simulink subsystem "PvtSubSys_VSM_HWA"  (R2020b)
settings: Solver=VariableStepAuto  StartTime=0.0  StopTime=10.0  RelTol=1e-3
values from neighbouring files (symbols this model uses):
  P_VSM_HWA_ALCStsSW = 1    [HWA.sldd]
  P_VSM_HWA_DMS_Enable = 0.0    [HWA.sldd]
  P_VSM_HWA_EHR_Enable = 0.0    [HWA.sldd]
  P_VSM_HWAActivation_NOAMOd_Spd = 5.0    [HWA.sldd]
  P_VSM_HWAActivation_Spd_Low = 5.0    [HWA.sldd]
  P_VSM_HWAActivation_Spd_Up = 120.0    [HWA.sldd]
  P_VSM_NOH_PilotSelc_SW = 0.0    [HWA.sldd]
  P_VSM_NOH_Swt_Req_SW = 0.0    [HWA.sldd]
  P_VSM_TJA_PassSBRSpdExistSlow = 30.0    [HWA.sldd]
undefined symbols (not defined in the file or in its folder): ACC_STATE, P_VSM_PassSBRSpdIPLimt, TJA_STATE
libraries: simulink x65, TrueDurationTime x14
(part 1 of 2)
settings Model: Creator=GW00133806  LastModifiedBy=GW00201299

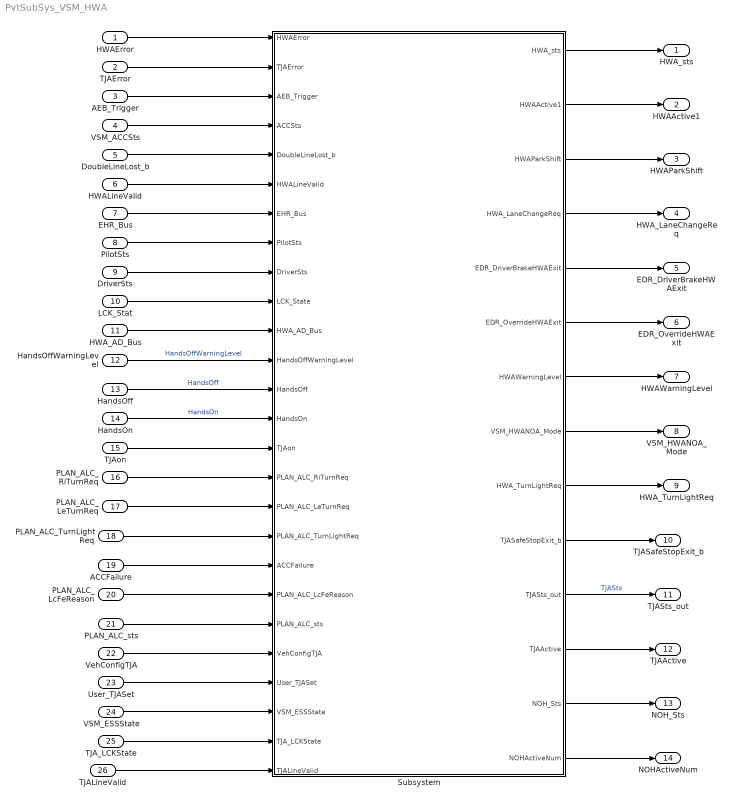
== system PvtSubSys_VSM_HWA ==
  HWAError : Inport  OutDataTypeStr=uint8
  TJAError : Inport  Port=2
  AEB_Trigger : Inport  Port=3  OutDataTypeStr=boolean
  VSM_ACCSts : Inport  Port=4  OutDataTypeStr=Enum: ACC_STATE
  DoubleLineLost_b : Inport  Port=5  OutDataTypeStr=boolean
  HWALineValid : Inport  Port=6  OutDataTypeStr=boolean
  EHR_Bus : Inport  Port=7  OutDataTypeStr=Bus: EHR_Bus
  PilotSts : Inport  Port=8  OutDataTypeStr=uint8
  DriverSts : Inport  Port=9  OutDataTypeStr=uint8
  LCK_Stat : Inport  Port=10
  HWA_AD_Bus : Inport  Port=11
  HandsOffWarningLevel : Inport  Port=12  OutDataTypeStr=uint8
  HandsOff : Inport  Port=13  OutDataTypeStr=boolean
  HandsOn : Inport  Port=14  OutDataTypeStr=boolean
  TJAon : Inport  Port=15  OutDataTypeStr=boolean
  PLAN_ALC_RiTurnReq : Inport  Port=16  OutDataTypeStr=uint8
  PLAN_ALC_LeTurnReq : Inport  Port=17  OutDataTypeStr=uint8
  PLAN_ALC_TurnLightReq : Inport  Port=18  OutDataTypeStr=uint8
  ACCFailure : Inport  Port=19
  PLAN_ALC_LcFeReason : Inport  Port=20
  PLAN_ALC_sts : Inport  Port=21
  VehConfigTJA : Inport  Port=22
  User_TJASet : Inport  Port=23
  VSM_ESSState : Inport  Port=24
  TJA_LCKState : Inport  Port=25
  TJALineValid : Inport  Port=26
  Subsystem : Subsystem
  HWA_sts : Outport  OutDataTypeStr=Enum: HWA_STATE
  HWAActive1 : Outport  Port=2  OutDataTypeStr=boolean
  HWAParkShift : Outport  Port=3  OutDataTypeStr=boolean
  HWA_LaneChangeReq : Outport  Port=4  OutDataTypeStr=uint8
  EDR_DriverBrakeHWAExit : Outport  Port=5  OutDataTypeStr=boolean
  EDR_OverrideHWAExit : Outport  Port=6  OutDataTypeStr=boolean
  HWAWarningLevel : Outport  Port=7  OutDataTypeStr=uint8
  VSM_HWANOA_Mode : Outport  Port=8  OutDataTypeStr=uint8
  HWA_TurnLightReq : Outport  Port=9
  TJASafeStopExit_b : Outport  Port=10
  TJASts_out : Outport  Port=11
  TJAActive : Outport  Port=12
  NOH_Sts : Outport  Port=13
  NOHActiveNum : Outport  Port=14
  wires:
  TJAError/1 -> Subsystem/2(TJAError)
  PLAN_ALC_sts/1 -> Subsystem/21(PLAN_ALC_sts)
  ACCFailure/1 -> Subsystem/19(ACCFailure)
  Subsystem/9(HWA_TurnLightReq) -> HWA_TurnLightReq/1
  PLAN_ALC_TurnLightReq/1 -> Subsystem/18(PLAN_ALC_TurnLightReq)
  Subsystem/8(VSM_HWANOA_Mode) -> VSM_HWANOA_Mode/1
  HandsOff/1 -> Subsystem/13(HandsOff)  "HandsOff"
  AEB_Trigger/1 -> Subsystem/3(AEB_Trigger)
  Subsystem/7(HWAWarningLevel) -> HWAWarningLevel/1
  Subsystem/5(EDR_DriverBrakeHWAExit) -> EDR_DriverBrakeHWAExit/1
  HWALineValid/1 -> Subsystem/6(HWALineValid)
  PilotSts/1 -> Subsystem/8(PilotSts)
  VSM_ACCSts/1 -> Subsystem/4(ACCSts)
  EHR_Bus/1 -> Subsystem/7(EHR_Bus)
  TJAon/1 -> Subsystem/15(TJAon)
  DoubleLineLost_b/1 -> Subsystem/5(DoubleLineLost_b)
  Subsystem/3(HWAParkShift) -> HWAParkShift/1
  Subsystem/2(HWAActive1) -> HWAActive1/1
  HandsOn/1 -> Subsystem/14(HandsOn)  "HandsOn"
  HWA_AD_Bus/1 -> Subsystem/11(HWA_AD_Bus)
  Subsystem/1(HWA_sts) -> HWA_sts/1
  PLAN_ALC_LeTurnReq/1 -> Subsystem/17(PLAN_ALC_LeTurnReq)
  LCK_Stat/1 -> Subsystem/10(LCK_State)
  DriverSts/1 -> Subsystem/9(DriverSts)
  HWAError/1 -> Subsystem/1(HWAError)
  Subsystem/6(EDR_OverrideHWAExit) -> EDR_OverrideHWAExit/1
  HandsOffWarningLevel/1 -> Subsystem/12(HandsOffWarningLevel)  "HandsOffWarningLevel"
  Subsystem/4(HWA_LaneChangeReq) -> HWA_LaneChangeReq/1
  PLAN_ALC_RiTurnReq/1 -> Subsystem/16(PLAN_ALC_RiTurnReq)
  PLAN_ALC_LcFeReason/1 -> Subsystem/20(PLAN_ALC_LcFeReason)
  VehConfigTJA/1 -> Subsystem/22(VehConfigTJA)
  User_TJASet/1 -> Subsystem/23(User_TJASet)
  VSM_ESSState/1 -> Subsystem/24(VSM_ESSState)
  TJA_LCKState/1 -> Subsystem/25(TJA_LCKState)
  TJALineValid/1 -> Subsystem/26(TJALineValid)
  Subsystem/10(TJASafeStopExit_b) -> TJASafeStopExit_b/1
  Subsystem/11(TJASts_out) -> TJASts_out/1  "TJASts"
  Subsystem/12(TJAActive) -> TJAActive/1
  Subsystem/13(NOH_Sts) -> NOH_Sts/1
  Subsystem/14(NOHActiveNum) -> NOHActiveNum/1

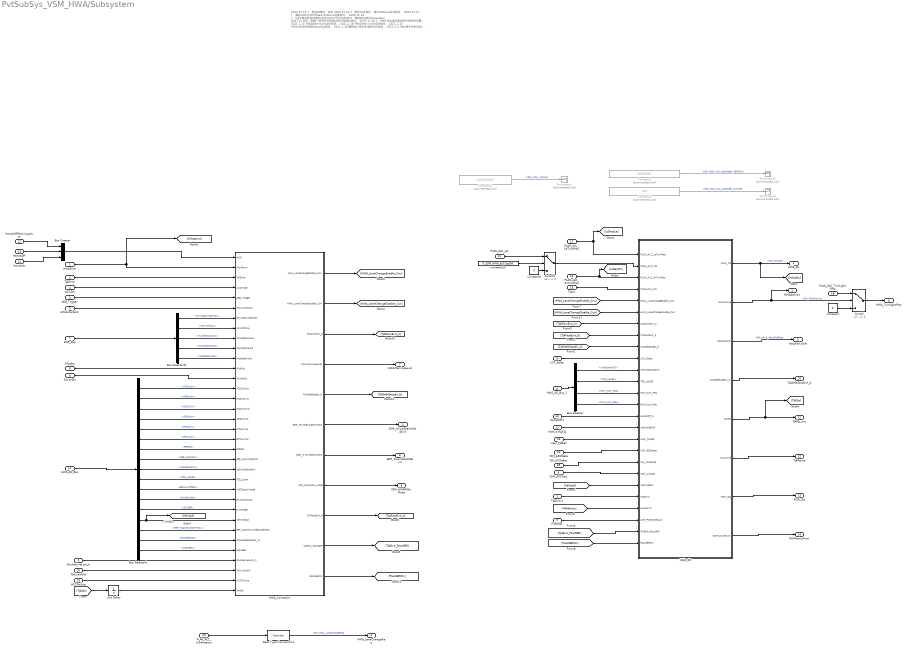
== system PvtSubSys_VSM_HWA/Subsystem ==
  note: 2020.12.15
      | 1、新框架释放，初版
      |
      | 2020.12.16
      | 1、更新NOA条件，增加NOAmode观测点；
      | 2020.12.17
      | 1、删除HWA状态机Ready到Active速度条件。
      | 2020.12.18
      | 1、HWA慢退进快退增加HWA状态处于CC校验条件，慢退条件满足且Handson
      |       且处于CC状态，屏蔽一些条件在换道过程中导致的退出。
      | 2020.12.28
      | 1. HWA 状态激活速度条件做成标定量。
      | 2021.1.15
      | HWAWarning状态机修改；
      | 2021.1.18
      | HWAWarning状态机修改；
      | 2021.1.19
      | HWA状态机换道信号coding修改；
      | 2021.1.20
      | 删除进入条件车速的时间校验；
      | 2021.2.2
      | HWA脱手条件连接。
      | 2021.2.5
      | HWA进慢退逻辑修改
      | 2021.2.6
      | 进慢退逻辑修改
      | 2021.2.8
      | 增加观测量；
      | 2021.2.17
      | 增加慢退条件ACCError
      | HWA状态机Error修改；
      | 2021.2.22
      | HWA_LaneChangeReq修改；
      | 接口修改；
      | 2021.2.26
      | 因PLAN版本未变更，断开ALCSts；
      | 2021.3.4
      | HWADriveOffConds修改HWA无法起步问题；
      | 2021.3.12
      | SafeStop置位延迟5s
      | 2021.3.13
      | 修改HWA跟停起步退出问题；
      | 解决HWA未激活报HWA_Warning的问题；
      | 2021.3.16
      | SingleLineLost进入慢退时加延时，增加标定量P_VSM_HWASlowExit_SingleLineLostDuring，默认3s；
  HWAError : Inport  OutDataTypeStr=uint8
  TJAError : Inport  Port=2
  AEB_Trigger : Inport  Port=3  OutDataTypeStr=boolean
  ACCSts : Inport  Port=4  OutDataTypeStr=Enum: ACC_STATE
  DoubleLineLost_b : Inport  Port=5
  HWALineValid : Inport  Port=6  OutDataTypeStr=boolean
  EHR_Bus : Inport  Port=7  OutDataTypeStr=Bus: EHR_Bus
  PilotSts : Inport  Port=8  OutDataTypeStr=uint8
  DriverSts : Inport  Port=9  OutDataTypeStr=uint8
  LCK_State : Inport  Port=10
  HWA_AD_Bus : Inport  Port=11
  HandsOffWarningLevel : Inport  Port=12  OutDataTypeStr=uint8
  HandsOff : Inport  Port=13  OutDataTypeStr=boolean
  HandsOn : Inport  Port=14  OutDataTypeStr=boolean
  TJAon : Inport  Port=15  OutDataTypeStr=boolean
  PLAN_ALC_RiTurnReq : Inport  Port=16  OutDataTypeStr=uint8
  PLAN_ALC_LeTurnReq : Inport  Port=17  OutDataTypeStr=uint8
  PLAN_ALC_TurnLightReq : Inport  Port=18
  ACCFailure : Inport  Port=19
  PLAN_ALC_LcFeReason : Inport  Port=20
  PLAN_ALC_sts : Inport  Port=21
  VehConfigTJA : Inport  Port=22
  User_TJASet : Inport  Port=23
  VSM_ESSState : Inport  Port=24
  TJA_LCKState : Inport  Port=25
  TJALineValid : Inport  Port=26
  Bus Creator : BusCreator  Inputs=3
  Bus Selector : BusSelector  OutputSignals=VehStandstill,TGS_LEVER,NOH_Swt_Req,NOH_Act_Req
  Bus Selector31 : BusSelector  OutputSignals=DrivingOnHighWay,FormOfWay,TunnelDistance,RampDistance,MapDataValid
  Bus Selector5 : BusSelector  OutputSignals=VDCActv,MSRActv,HDCCtrl,ABSActv,PTCActv,BTCActv,EPBSts,EPB_SwtPosn,VehStandstill,TGS_LEVER,ESPFuncOffSts,DrvDoorSts,DrvSBR,VehSpd,ESP_MasterCylBrkPress,BrkPedalSts,PassSBR
  Constant : Constant  Value=0  OutDataTypeStr=uint8
  Constant1 : Constant  Commented=on  Value=38260536  OutDataTypeStr=uint32
  Constant10 : Constant  Value=P_VSM_HWA_ALCStsSW
  Constant2 : Constant  Commented=on  Value=2103160605
  Constant3 : Constant  Commented=on  Value=301  OutDataTypeStr=uint16
  Constant9 : Constant  Value=0  OutDataTypeStr=uint8
  Data Type Conversion1 : DataTypeConversion
  HWA_AD_Bus_1 : InportShadow  Port=11
  HWA_Condotion : Subsystem
  HWA_SM : Subsystem
  HandsOff1 : InportShadow  Port=13  OutDataTypeStr=boolean
  PilotSts1 : InportShadow  Port=8  OutDataTypeStr=uint8
  Switch : Switch  Criteria=u2 ~= 0
  Switch6 : Switch  Criteria=u2 ~= 0
  TJAError1 : InportShadow  Port=2
  Terminator1 : Terminator  Commented=on
  Terminator2 : Terminator  Commented=on
  Terminator3 : Terminator  Commented=on
  Unit Delay : UnitDelay  InitialCondition=TJA_STATE.TJA_Off  SampleTime=-1  HasFrameUpgradeWarning=on
  VSM_ACCSts1 : InportShadow  Port=4  OutDataTypeStr=Enum: ACC_STATE
  HWA_sts : Outport  OutDataTypeStr=Enum: HWA_STATE
  HWAActive1 : Outport  Port=2  OutDataTypeStr=boolean
  HWAParkShift : Outport  Port=3  OutDataTypeStr=boolean
  HWA_LaneChangeReq : Outport  Port=4  OutDataTypeStr=uint8
  EDR_DriverBrakeHWAExit : Outport  Port=5  OutDataTypeStr=boolean
  EDR_OverrideHWAExit : Outport  Port=6  OutDataTypeStr=boolean
  HWAWarningLevel : Outport  Port=7  OutDataTypeStr=uint8
  VSM_HWANOA_Mode : Outport  Port=8  OutDataTypeStr=uint8
  HWA_TurnLightReq : Outport  Port=9
  TJASafeStopExit_b : Outport  Port=10
  TJASts_out : Outport  Port=11
  TJAActive : Outport  Port=12
  NOH_Sts : Outport  Port=13
  NOHActiveNum : Outport  Port=14
  wires:
  [TJAExit_PassSBR] -> HWA_SM/25(TJAExit_PassSBR)
  [PassSBROn] -> HWA_SM/26(PassSBROn)
  HWA_Condotion/11(PassSBROn) -> [PassSBROn]
  HWA_Condotion/10(TJAExit_PassSBR) -> [TJAExit_PassSBR]
  Bus Selector5/17 -> HWA_Condotion/30("PassSBR ")  "<PassSBR>"
  HWA_SM/8(NOHActiveNum) -> NOHActiveNum/1
  Bus Selector/4 -> HWA_SM/14(NOH_Act_Req)  "<NOH_Act_Req>"
  HWA_SM/7(NOH_Sts) -> NOH_Sts/1
  Bus Selector/3 -> HWA_SM/13(NOH_Swt_Req)  "<NOH_Swt_Req>"
  PilotSts1/1 -> HWA_SM/24(LSM_PilotModeCalc)
  [HWAerror] -> HWA_SM/23(HWAerror)
  HWA_SM/6(TJAActive) -> TJAActive/1
  [VehSpd] -> HWA_SM/21(VehicleSpd)
  Unit Delay/1 -> HWA_Condotion/34(TJASts)
  [TJASts] -> Unit Delay/1
  TJALineValid/1 -> HWA_Condotion/32(TJALineValid)
  DoubleLineLost_b/1 -> HWA_Condotion/31(DoubleLineLost_b)
  TJA_LCKState/1 -> HWA_SM/19(TJA_LCKState)
  VSM_ESSState/1 -> HWA_SM/18(VSM_ESSState)
  User_TJASet/1 -> HWA_SM/17(User_TJASet)
  VehConfigTJA/1 -> HWA_SM/16(VehConfigTJA)
  VSM_ACCSts1/1 -> HWA_SM/20(VSM_ACCSts)
  HandsOff1/1 -> HWA_SM/15(HandsOff_b)
  HWA_SM/5(TJASts) -> TJASts_out/1, [TJASts]
  HWA_SM/4(TJASafeStopExit_b) -> TJASafeStopExit_b/1
  [TJASafeStopEn_b] -> HWA_SM/9(TJASafeStopEn_b)
  [TJAFastExit_b] -> HWA_SM/8(TJAFastExit_b)
  HWA_Condotion/9(TJAFastExit_b) -> [TJAFastExit_b]
  HWALineValid/1 -> HWA_Condotion/6(HWALineValid)
  Bus Selector5/15 -> HWA_Condotion/28(ESP_MasterCylindBrakePress)  "<ESP_MasterCylBrkPress>"
  HWA_SM/1(HWA_sts) -> [HWASts], HWA_sts/1  "VSM_HWASts"
  DriverSts/1 -> HWA_Condotion/13(DriverSts)
  Bus Selector31/1 -> HWA_Condotion/7(DrivingOnHighWay)  "<DrivingOnHighWay>"
  HWA_Condotion/2(HWA_LaneChangeDisable_Con) -> [HWA_LaneChangeDisable_Con]
  Bus Selector5/10 -> HWA_Condotion/23(TGS_Lever)  "<TGS_LEVER>"
  HWA_SM/2(HWAActive) -> Switch/2, HWAActive1/1  "VSM_HWAActive"
  Bus Selector5/3 -> HWA_Condotion/16(HDCControl)  "<HDCCtrl>"
  PilotSts/1 -> HWA_Condotion/12(PilotSts)
  AEB_Trigger/1 -> HWA_Condotion/5(AEB_Trigger)
  Bus Selector5/9 -> HWA_Condotion/22(VehicleStandstill)  "<VehStandstill>"
  PLAN_ALC_RiTurnReq/1 -> HWA_SM/3(PLAN_ALC_RiTurnReq), [LcDecsRi]
  HWA_AD_Bus/1 -> Bus Selector5/1
  Bus Selector5/16 -> HWA_Condotion/29(BrakePedalStatus_G)  "<BrkPedalSts>"
  Bus Selector5/1 -> HWA_Condotion/14(VDCActive)  "<VDCActv>"
  HWA_SM/3(TJAParkShift) -> HWAParkShift/1  "VSM_HWA_ParkShiftReq"
  HWAError/1 -> HWA_Condotion/2(HWAError), [HWAerror]
  Bus Creator/1 -> HWA_Condotion/1(HOD)
  Bus Selector5/7 -> HWA_Condotion/20(EPBSts)  "<EPBSts>"
  HWA_AD_Bus_1/1 -> Bus Selector/1
  [HWA_LaneChangeDisable_Con] -> HWA_SM/6(HWA_LaneChangeDisable_Con)
  HandsOffWarningLevel/1 -> Bus Creator/1
  HWA_Condotion/1(HWA_LaneChangeEnable_Con) -> [HWA_LaneChangeEnable_Con]
  Bus Selector5/2 -> HWA_Condotion/15(MSRActive)  "<MSRActv>"
  [HWA_LaneChangeEnable_Con] -> HWA_SM/5(HWA_LaneChangeEnable_Con)
  Bus Selector5/12 -> HWA_Condotion/25(DriverDoorSts)  "<DrvDoorSts>"
  HWA_Condotion/6(EDR_DriverBrakeHWAExit) -> EDR_DriverBrakeHWAExit/1
  TJAon/1 -> HWA_SM/4(TJASwitch_ON)
  Bus Selector31/4 -> HWA_Condotion/10(RampDistance)  "<RampDistance>"
  EHR_Bus/1 -> Bus Selector31/1
  HandsOff/1 -> Bus Creator/2
  Bus Selector5/11 -> HWA_Condotion/24(VDCDeactivated)  "<ESPFuncOffSts>"
  Bus Selector5/14 -> HWA_Condotion/27(VehicleSpd), [VehSpd]  "<VehSpd>"
  HandsOn/1 -> Bus Creator/3
  HWA_Condotion/4(HWAWarningLevel) -> HWAWarningLevel/1
  Bus Selector5/5 -> HWA_Condotion/18(PTCActive)  "<PTCActv>"
  [TJASlowExit_b] -> HWA_SM/7(TJASlowExit_b)
  HWA_Condotion/3(TJASlowExit_b) -> [TJASlowExit_b]
  Bus Selector5/13 -> HWA_Condotion/26(DriverSBR)  "<DrvSBR>"
  Bus Selector/1 -> HWA_SM/11(VehicleStandstill)  "<VehStandstill>"
  Bus Selector5/4 -> HWA_Condotion/17(ABSActive)  "<ABSActv>"
  Bus Selector31/2 -> HWA_Condotion/8(FormOfWay)  "<FormOfWay>"
  HWA_Condotion/5(TJASafeStopEn_b) -> [TJASafeStopEn_b]
  Bus Selector31/3 -> HWA_Condotion/9(TunnelDistance)  "<TunnelDistance>"
  Bus Selector5/8 -> HWA_Condotion/21(EPB_SwtichPositon)  "<EPB_SwtPosn>"
  Bus Selector5/6 -> HWA_Condotion/19(BTCActive)  "<BTCActv>"
  PLAN_ALC_LeTurnReq/1 -> [LcDecsLe], HWA_SM/1(PLAN_ALC_LeTurnReq)
  Bus Selector31/5 -> HWA_Condotion/11(MapDataValid)  "<MapDataValid>"
  LCK_State/1 -> HWA_SM/10(LCK_State)
  HWA_Condotion/7(EDR_OverrideHWAExit) -> EDR_OverrideHWAExit/1
  ACCSts/1 -> HWA_Condotion/4(ACCMode)
  Data Type Conversion1/1 -> HWA_LaneChangeReq/1  "VSM_HWA_LaneChangeReq"
  HWA_Condotion/8(VSM_HWANOA_Mode) -> VSM_HWANOA_Mode/1
  PLAN_ALC_TurnLightReq/1 -> Switch/1
  Constant/1 -> Switch/3
  Switch/1 -> HWA_TurnLightReq/1
  Constant2/1 -> Terminator1/1  "VSM_HWA_Version"
  ACCFailure/1 -> HWA_Condotion/33(ACCFailure)
  Switch6/1 -> HWA_SM/2(PLAN_ALC_sts)
  Constant10/1 -> Switch6/2
  Constant9/1 -> Switch6/3
  PLAN_ALC_sts/1 -> Switch6/1
  PLAN_ALC_LcFeReason/1 -> Data Type Conversion1/1
  Bus Selector/2 -> HWA_SM/12(TGS_LEVER)  "<TGS_LEVER>"
  TJAError/1 -> HWA_Condotion/3(TJAError)
  TJAError1/1 -> HWA_SM/22(TJAError)
  Constant3/1 -> Terminator3/1  "VSM_HWA_TJA_SubModel_Number"
  Constant1/1 -> Terminator2/1  "VSM_HWA_TJA_SubModel_VERSION"

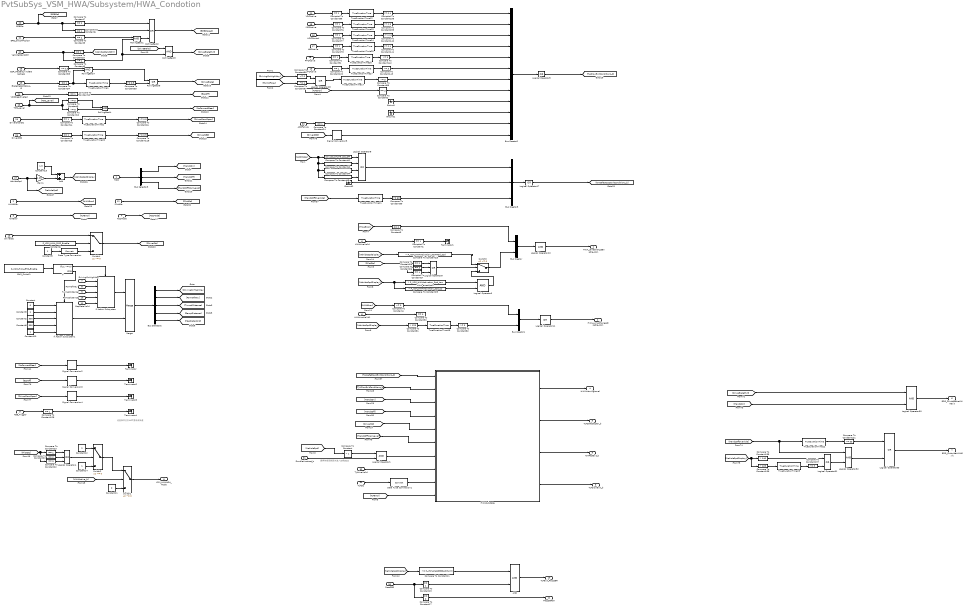
== system PvtSubSys_VSM_HWA/Subsystem/HWA_Condotion ==
  note: 跟停时报双侧丢失进入safestop
  note: 这些条件已在ACC里设成快退
  HOD : Inport
  HWAError : Inport  Port=2
  TJAError : Inport  Port=3
  ACCMode : Inport  Port=4
  AEB_Trigger : Inport  Port=5
  HWALineValid : Inport  Port=6
  DrivingOnHighWay : Inport  Port=7
  FormOfWay : Inport  Port=8
  TunnelDistance : Inport  Port=9
  RampDistance : Inport  Port=10
  MapDataValid : Inport  Port=11
  PilotSts : Inport  Port=12
  DriverSts : Inport  Port=13
  VDCActive : Inport  Port=14
  MSRActive : Inport  Port=15
  HDCControl : Inport  Port=16
  ABSActive : Inport  Port=17
  PTCActive : Inport  Port=18
  BTCActive : Inport  Port=19
  EPBSts : Inport  Port=20
  EPB_SwtichPositon : Inport  Port=21
  VehicleStandstill : Inport  Port=22
  TGS_Lever : Inport  Port=23
  VDCDeactivated : Inport  Port=24
  DriverDoorSts : Inport  Port=25
  DriverSBR : Inport  Port=26
  VehicleSpd : Inport  Port=27
  ESP_MasterCylindBrakePress : Inport  Port=28
  BrakePedalStatus_G : Inport  Port=29
  "PassSBR " : Inport  Port=30
  DoubleLineLost_b : Inport  Port=31
  TJALineValid : Inport  Port=32
  ACCFailure : Inport  Port=33
  TJASts : Inport  Port=34
  AND : Logic  AllPortsSameDT=off  OutDataTypeStr=boolean
  Add : Sum
  Bus Creator : BusCreator  Inputs=2
  Bus Creator1 : BusCreator  Inputs=2
  Bus Creator5 : BusCreator  Inputs=3
  Bus Selector2 : BusSelector  OutputSignals=DrivingOnHighWay,FormOfWay,TunnelDistance,RampDistance,MapDataValid
  Bus Selector3 : BusSelector  OutputSignals=HandsOn,HandsOff,HandsOffWarningLevel
  Bus Creator2 : BusCreator  Inputs=12
  Compare To Constant : simulink/Logic and Bit Operations/Compare To Constant  relop=>  const=1  OutDataTypeStr=boolean
  Compare To Constant11 : simulink/Logic and Bit Operations/Compare To Constant  relop=>=  const=P_VSM_PassSBRSpdIPLimt  OutDataTypeStr=boolean
  Compare To Constant{1,6,12..15,19,23..24,34,56,76..78,91,120,128} (17 alike) : simulink/Logic and Bit Operations/Compare To Constant  relop===  const=1  OutDataTypeStr=boolean
  Compare To Constant17 : simulink/Logic and Bit Operations/Compare To Constant  relop===  const=0  OutDataTypeStr=boolean
  Compare To Constant2 : simulink/Logic and Bit Operations/Compare To Constant  relop===  const=3  OutDataTypeStr=boolean
  Compare To Constant10 : simulink/Logic and Bit Operations/Compare To Constant  relop=~=  const=8  OutDataTypeStr=boolean
  Compare To Constant{16,33,35,118} (4 alike) : simulink/Logic and Bit Operations/Compare To Constant  relop=>=  const=0.5  OutDataTypeStr=boolean
  Compare To Constant121 : simulink/Logic and Bit Operations/Compare To Constant  relop=>=  const=60  OutDataTypeStr=boolean
  Compare To Constant135 : simulink/Logic and Bit Operations/Compare To Constant  relop=>  const=140  OutDataTypeStr=boolean
  Compare To Constant136 : simulink/Logic and Bit Operations/Compare To Constant  relop=>  const=125  OutDataTypeStr=boolean
  Compare To Constant{82,137,142..143} (4 alike) : simulink/Logic and Bit Operations/Compare To Constant  relop=>=  const=3  OutDataTypeStr=boolean
  Compare To Constant138 : simulink/Logic and Bit Operations/Compare To Constant  relop=>=  const=0.4  OutDataTypeStr=boolean
  Compare To Constant139 : simulink/Logic and Bit Operations/Compare To Constant  relop=>=  const=0.8  OutDataTypeStr=boolean
  Compare To Constant140 : simulink/Logic and Bit Operations/Compare To Constant  relop=>=  const=0.04  OutDataTypeStr=boolean
  Compare To Constant141 : simulink/Logic and Bit Operations/Compare To Constant  relop=>=  const=0.4  OutDataTypeStr=boolean
  Compare To Constant{7..8,21,28} (4 alike) : simulink/Logic and Bit Operations/Compare To Constant  relop===  const=2  OutDataTypeStr=boolean
  Compare To Constant22 : simulink/Logic and Bit Operations/Compare To Constant  relop===  const=3  OutDataTypeStr=boolean
  Compare To Constant25 : simulink/Logic and Bit Operations/Compare To Constant  relop=>  const=P_VSM_HWAActivation_NOAMOd_Spd  OutDataTypeStr=boolean
  Compare To Constant26 : simulink/Logic and Bit Operations/Compare To Constant  relop===  const=3  OutDataTypeStr=boolean
  Compare To Constant27 : simulink/Logic and Bit Operations/Compare To Constant  relop===  const=4  OutDataTypeStr=boolean
  Compare To Constant29 : simulink/Logic and Bit Operations/Compare To Constant  relop=<  const=P_VSM_HWAActivation_Spd_Up  OutDataTypeStr=boolean
  Compare To Constant3 : simulink/Logic and Bit Operations/Compare To Constant  relop===  const=0  OutDataTypeStr=boolean
  Compare To Constant30 : simulink/Logic and Bit Operations/Compare To Constant  relop===  const=0  OutDataTypeStr=boolean
  Compare To Constant39 : simulink/Logic and Bit Operations/Compare To Constant  relop=>=  const=60  OutDataTypeStr=boolean
  Compare To Constant4 : simulink/Logic and Bit Operations/Compare To Constant  relop=~=  const=0  OutDataTypeStr=boolean
  Compare To Constant41 : simulink/Logic and Bit Operations/Compare To Constant  relop===  const=ACC_STATE.ACC_Off  OutDataTypeStr=boolean
  Compare To Constant42 : simulink/Logic and Bit Operations/Compare To Constant  relop===  const=ACC_STATE.ACC_Reject  OutDataTypeStr=boolean
  Compare To Constant44 : simulink/Logic and Bit Operations/Compare To Constant  relop===  const=ACC_STATE.ACC_Standby  OutDataTypeStr=boolean
  Compare To Constant45 : simulink/Logic and Bit Operations/Compare To Constant  relop===  const=ACC_STATE.ACC_Failure  OutDataTypeStr=boolean
  Compare To Constant5 : simulink/Logic and Bit Operations/Compare To Constant  relop=~=  const=1  OutDataTypeStr=boolean
  Compare To Constant81 : simulink/Logic and Bit Operations/Compare To Constant  relop=>  const=125  OutDataTypeStr=boolean
  Compare To Constant86 : simulink/Logic and Bit Operations/Compare To Constant  relop=~=  const=0  OutDataTypeStr=boolean
  Compare To Constant87 : simulink/Logic and Bit Operations/Compare To Constant  relop=~=  const=1  OutDataTypeStr=boolean
  Compare To Constant88 : simulink/Logic and Bit Operations/Compare To Constant  relop=>=  const=5  OutDataTypeStr=boolean
  Compare To Constant9 : simulink/Logic and Bit Operations/Compare To Constant  relop=~=  const=5  OutDataTypeStr=boolean
  Constant : Constant  Value=0  OutDataTypeStr=Inherit: Inherit via back propagation
  Constant10 : Constant  OutDataTypeStr=Inherit: Inherit via back propagation
  Constant11 : Constant  Value=0  OutDataTypeStr=uint8
  Constant12 : Constant  Value=2  OutDataTypeStr=uint8
  Constant13 : Constant  Value=1.3
  Constant14 : Constant  OutDataTypeStr=uint8
  Constant2 : Constant  Value=500  OutDataTypeStr=Inherit: Inherit via back propagation
  Constant3 : Constant  OutDataTypeStr=Inherit: Inherit via back propagation
  Constant6 : Constant  Value=P_VSM_HWA_DMS_Enable
  Constant8 : Constant  Value=500  OutDataTypeStr=Inherit: Inherit via back propagation
  Constant9 : Constant
  Data Type Conversion : DataTypeConversion
  Data Type Conversion1 : DataTypeConversion
  EHR_Switch1 : Constant  Value=P_VSM_HWA_EHR_Enable
  Gain1 : Gain  Gain=1.03
  Ground : Ground
  Ground1 : Ground
  Ground2 : Ground
  HWALineValid1 : InportShadow  Port=6
  HWASubstate : Stateflow chart  TreatAsAtomicUnit=on
  HWA_enterSpd1 : simulink/Logic and Bit Operations/Compare To Constant  relop=>  const=P_VSM_HWAActivation_Spd_Low  OutDataTypeStr=boolean
  If : If  IfExpression=u1 ~= 0
  If Action Subsystem : Subsystem  TreatAsAtomicUnit=on
  If Action Subsystem1 : Subsystem  TreatAsAtomicUnit=on
  Logical Operator{1,6,30,32} (4 alike) : Logic  AllPortsSameDT=off  OutDataTypeStr=boolean
  Logical Operator10 : Logic  Inputs=1  AllPortsSameDT=off  OutDataTypeStr=boolean
  Logical Operator11 : Logic  Operator=OR  Inputs=1  AllPortsSameDT=off  OutDataTypeStr=boolean
  Logical Operator17 : Logic  Operator=OR  Inputs=1  AllPortsSameDT=off  OutDataTypeStr=boolean
  Logical Operator18 : Logic  Operator=OR  AllPortsSameDT=off  OutDataTypeStr=boolean
  Logical Operator31 : Logic  Operator=OR  AllPortsSameDT=off  OutDataTypeStr=boolean
  Logical Operator33 : Logic  Operator=OR  AllPortsSameDT=off  OutDataTypeStr=boolean
  Logical Operator4 : Logic  Operator=OR  Inputs=3  AllPortsSameDT=off  OutDataTypeStr=boolean
  Logical Operator5 : Logic  Operator=OR  Inputs=1  AllPortsSameDT=off  OutDataTypeStr=boolean
  Logical Operator8 : Logic  Operator=OR  Inputs=4  AllPortsSameDT=off  OutDataTypeStr=boolean
  Logical Operator9 : Logic  Operator=OR  Inputs=3  AllPortsSameDT=off  OutDataTypeStr=boolean
  Merge : Merge
  RollingBack{1,3..4,7} (4 alike) : Logic  AllPortsSameDT=off  OutDataTypeStr=boolean
  RollingBack2 : Logic  Operator=OR  Inputs=3  AllPortsSameDT=off  OutDataTypeStr=boolean
  RollingBack8 : Logic  Operator=OR  AllPortsSameDT=off  OutDataTypeStr=boolean
  Signal Conversion{2..5} (4 alike) : SignalConversion  OverrideOpt=off
  Switch{1..4} (4 alike) : Switch  Criteria=u2 ~= 0
  Terminator{,1..4} (5 alike) : Terminator
  TrueDurationTime{1..2,11..13,15,17,20,22..27} (14 alike) : TrueDurationTime/TrueDurationTime  TCycle=0.02
  HWA_LaneChangeEnable_Con : Outport
  HWA_LaneChangeDisable_Con : Outport  Port=2
  TJASlowExit_b : Outport  Port=3
  HWAWarningLevel : Outport  Port=4
  TJASafeStopEn_b : Outport  Port=5
  EDR_DriverBrakeHWAExit : Outport  Port=6
  EDR_OverrideHWAExit : Outport  Port=7
  VSM_HWANOA_Mode : Outport  Port=8
  TJAFastExit_b : Outport  Port=9
  TJAExit_PassSBR : Outport  Port=10
  PassSBROn : Outport  Port=11
  wires:
  Compare To Constant17/1 -> PassSBROn/1
  AND/1 -> TJAExit_PassSBR/1
  Compare To Constant13/1 -> AND/2
  Compare To Constant11/1 -> AND/1
  [VehicleSpdDisplay] -> Compare To Constant11/1
  "PassSBR "/1 -> Compare To Constant13/1, Compare To Constant17/1
  Compare To Constant1/1 -> Terminator1/1
  Data Type Conversion1/1 -> HWASubstate/9(TJASts)
  TJASts/1 -> Data Type Conversion1/1
  TJALineValid/1 -> HWASubstate/8(TJALineValid)
  DoubleLineLost_b/1 -> Logical Operator1/2
  [VehicleSpdDisplay] -> Compare To Constant81/1
  Compare To Constant82/1 -> Bus Creator1/2
  TrueDurationTime15/1 -> Compare To Constant82/1
  Compare To Constant81/1 -> TrueDurationTime15/1
  HWALineValid1/1 -> Compare To Constant30/1
  Logical Operator11/1 -> HWA_LaneChangeDisable_Con/1  "VSM_HWA_LaneChangeDisable_Con"
  Bus Creator1/1 -> Logical Operator11/1
  Logical Operator10/1 -> HWA_LaneChangeEnable_Con/1  "VSM_HWA_LaneChangeEnable_Con"
  Bus Creator/1 -> Logical Operator10/1
  Switch3/1 -> Bus Creator/2
  Compare To Constant27/1 -> Logical Operator9/3
  [VehicleSpdDisplay] -> HWA_enterSpd1/1, Compare To Constant29/1
  Logical Operator9/1 -> Switch3/2
  Compare To Constant28/1 -> Logical Operator9/1
  [PilotSts] -> Compare To Constant27/1, Compare To Constant26/1, Compare To Constant28/1
  Logical Operator6/1 -> Switch3/3
  Compare To Constant26/1 -> Logical Operator9/2
  Compare To Constant29/1 -> Logical Operator6/2
  HWA_enterSpd1/1 -> Logical Operator6/1
  Compare To Constant25/1 -> Switch3/1
  [VehicleSpdDisplay] -> Compare To Constant25/1
  HWALineValid/1 -> Compare To Constant1/1
  [DriveBrakeExit] -> Logical Operator30/1
  ACCMode/1 -> [ACCMode]
  ESP_MasterCylindBrakePress/1 -> Compare To Constant33/1
  RollingBack8/1 -> [DriveBrake]
  Compare To Constant34/1 -> RollingBack7/2, TrueDurationTime1/1
  Compare To Constant33/1 -> RollingBack7/1
  RollingBack7/1 -> RollingBack8/1
  BrakePedalStatus_G/1 -> Compare To Constant34/1
  Compare To Constant35/1 -> RollingBack8/2
  TrueDurationTime1/1 -> Compare To Constant35/1
  Add/1 -> [VehicleSpdDisplay]
  Constant13/1 -> Add/1
  VehicleSpd/1 -> Gain1/1, [VehicleSpd]
  Gain1/1 -> Add/2
  DriverSBR/1 -> Compare To Constant15/1
  TrueDurationTime2/1 -> Compare To Constant16/1
  DriverDoorSts/1 -> Compare To Constant14/1
  Compare To Constant14/1 -> TrueDurationTime2/1
  Compare To Constant118/1 -> [DriverSBR]  "DriverSBR"
  Compare To Constant15/1 -> TrueDurationTime20/1
  Compare To Constant16/1 -> [DriverDoorOpen]  "DriverDoorOpen"
  TrueDurationTime20/1 -> Compare To Constant118/1
  VDCDeactivated/1 -> Compare To Constant12/1
  Compare To Constant12/1 -> [EspOff]  "EspOff"
  EPBSts/1 -> Compare To Constant7/1, Compare To Constant6/1, [EPBSts]
  Compare To Constant6/1 -> RollingBack2/2
  Compare To Constant5/1 -> RollingBack1/2, RollingBack3/2
  Compare To Constant7/1 -> RollingBack2/1
  VehicleStandstill/1 -> Compare To Constant5/1, Compare To Constant19/1
  EPB_SwtichPositon/1 -> Compare To Constant8/1
  TGS_Lever/1 -> Compare To Constant10/1, Compare To Constant9/1, [TGS_Lever]
  RollingBack2/1 -> [EPBClosed]  "EPBClosed"
  Compare To Constant10/1 -> RollingBack4/2
  Compare To Constant9/1 -> RollingBack4/1
  Compare To Constant19/1 -> [VehicleStandStill]
  RollingBack3/1 -> [DriveBrakeExit]  "DriverBrakeExit"
  [DriveBrake] -> RollingBack3/1
  RollingBack4/1 -> [NoForwardGear]  "NoForwardGear"
  Compare To Constant8/1 -> RollingBack1/1
  RollingBack1/1 -> RollingBack2/3
  [FormOfWay] -> Compare To Constant87/1
  Constant/1 -> If Action Subsystem1/1(In1)  "DrivingOnHighWay"
  HWASubstate/1(HWAWarningLevel) -> HWAWarningLevel/1  "VSM_HWAWarningLevel"
  [TJAError] -> Compare To Constant2/1
  Compare To Constant88/1 -> Bus Creator2/7  "VSM_HWASlowExitCons_NotHighWayArterialRoad5s"
  Compare To Constant41/1 -> Logical Operator8/1
  FormOfWay/1 -> If Action Subsystem/2(In2)
  TrueDurationTime11/1 -> Compare To Constant39/1
  [DriverSts] -> HWASubstate/5(DriverSts)
  Ground1/1 -> Bus Creator2/10  "VSM_HWASlowExitCons_HWAError_ErrorBlindness"
  [HandsOff] -> HWASubstate/4(HandsOff_b)  "VSM_HandsOff"
  [HandsOn] -> HWASubstate/3(HandsOn_b)  "VSM_HandsOn"
  Bus Selector2/5 -> [MapDataValid]  "<MapDataValid>"
  Ground/1 -> Bus Creator2/9  "VSM_HWASlowExitCons_HWAError_Error"
  [TJASlowExitConditions_b] -> HWASubstate/2(TJASlowExitConditions_b)
  AEB_Trigger/1 -> Compare To Constant128/1
  HWASubstate/2(TJASafeStopEn_b) -> TJASafeStopEn_b/1  "VSM_HWASafeStopEn"
  Constant6/1 -> Switch4/2
  Compare To Constant128/1 -> Terminator4/1  "VSM_HWASlowExitCons_AEBTrigger"
  Bus Creator5/1 -> Logical Operator17/1  "SomeHWASafeStop2ExitConds"
  Compare To Constant86/1 -> Logical Operator18/1
  Logical Operator32/1 -> Logical Operator33/2  "SpeedTooHighWithOverride"
  [TJASafeStop2ExitConditions_b] -> HWASubstate/1(SomeHWASafeStop2ExitConditions_b)
  Compare To Constant135/1 -> Logical Operator31/1
  TrueDurationTime24/1 -> Compare To Constant140/1
  [DriverSBR] -> Signal Conversion5/1
  MSRActive/1 -> Compare To Constant76/1
  [DriverDoorOpen] -> Signal Conversion4/1
  TunnelDistance/1 -> If Action Subsystem/3(TunnelDistance)
  Signal Conversion4/1 -> Terminator3/1  "VSM_HWASlowExitCons_DriverDoorOpen"
  Compare To Constant45/1 -> Logical Operator8/4
  Logical Operator30/1 -> EDR_DriverBrakeHWAExit/1  "EDR_DriverBrakeHWAExit"
  [HandsOffOverride] -> TrueDurationTime22/1, Logical Operator32/1
  Compare To Constant136/1 -> TrueDurationTime23/1
  TrueDurationTime23/1 -> Compare To Constant137/1
  [HandsOffOverride] -> TrueDurationTime11/1
  Signal Conversion3/1 -> Terminator2/1  "VSM_HWASlowExitCons_ESPOff"
  [HandsOffWarnLevel] -> HWASubstate/6(HandsOffWarnLevel)
  Data Type Conversion/1 -> Switch4/3
  Bus Creator2/1 -> Logical Operator5/1  "HWASlowExitConditions"
  Compare To Constant87/1 -> Logical Operator18/2
  Bus Selector3/2 -> [HandsOff]  "<HandsOff>"
  Bus Selector2/2 -> [FormOfWay]  "<FormOfWay>"
  DriverSts/1 -> Switch4/1
  MapDataValid/1 -> If Action Subsystem/5(MapDataValid)
  HWAError/1 -> [HWAError]  "VSM_Diagnostic_HWAError"
  Ground2/1 -> Bus Creator5/2  "VSM_HWAFastExitCons_HWAErrorFastExit"
  TrueDurationTime27/1 -> Compare To Constant143/1
  TrueDurationTime25/1 -> Compare To Constant141/1
  BTCActive/1 -> Compare To Constant120/1
  HWASubstate/4(TJASlowExit_b) -> TJASlowExit_b/1  "VSM_HWASlowExit_b"
  Compare To Constant142/1 -> Bus Creator2/5  "VSM_HWASlowExitCons_TCS1Active3000ms"
  Compare To Constant140/1 -> Bus Creator2/3  "VSM_HWASlowExitCons_HDCActive40ms"
  Compare To Constant42/1 -> Logical Operator8/2
  Compare To Constant141/1 -> Bus Creator2/4  "VSM_HWASlowExitCons_ABSActive400ms"
  If Action Subsystem/1(Out1) -> Merge/1
  Constant9/1 -> Data Type Conversion/1
  Compare To Constant56/1 -> TrueDurationTime12/1
  Bus Selector3/3 -> [HandsOffWarnLevel]  "<HandsOffWarningLevel>"
  DrivingOnHighWay/1 -> If Action Subsystem/1(In1)
  Bus Selector3/1 -> [HandsOn]  "<HandsOn>"
  Compare To Constant78/1 -> TrueDurationTime25/1
  [ACCMode] -> Compare To Constant44/1, Compare To Constant45/1, Compare To Constant42/1, Compare To Constant41/1
  Logical Operator33/1 -> EDR_OverrideHWAExit/1  "EDR_OverrideHWAExit"
  Logical Operator31/1 -> Logical Operator32/2
  Compare To Constant91/1 -> TrueDurationTime26/1
  Logical Operator17/1 -> [TJASafeStop2ExitConditions_b]  "VSM_SomeHWASafeStop2ExitConditions_b"
  Bus Selector2/1 -> [DrivingOnHighWay]  "<DrivingOnHighWay>"
  Switch4/1 -> [DriverSts]  "DriverSts"
  [VehicleSpdDisplay] -> Compare To Constant136/1, Compare To Constant135/1
  TrueDurationTime12/1 -> Compare To Constant138/1
  Logical Operator5/1 -> [TJASlowExitConditions_b]  "VSM_HWASlowExitConditions_b"
  [EspOff] -> Signal Conversion3/1
  Compare To Constant120/1 -> TrueDurationTime27/1
  Constant2/1 -> If Action Subsystem1/3(In3)  "TunnelDistance"
  [NoForwardGear] -> Signal Conversion2/1
  ABSActive/1 -> Compare To Constant78/1
  VDCActive/1 -> Compare To Constant56/1
  Signal Conversion2/1 -> Terminator/1  "VSM_HWASlowExitCons_NoForwardGear"
  PilotSts/1 -> [PilotSts]
  Signal Conversion5/1 -> Bus Creator2/12  "VSM_HWAFastExitCons_DriverSBR"
  TrueDurationTime13/1 -> Compare To Constant139/1
  TrueDurationTime17/1 -> Compare To Constant88/1
  Compare To Constant138/1 -> Bus Creator2/1  "VSM_HWASlowExitCons_EspActive400ms"
  TrueDurationTime26/1 -> Compare To Constant142/1
  Bus Selector2/3 -> [TunnelDistance]  "<TunnelDistance>"
  PTCActive/1 -> Compare To Constant91/1
  Compare To Constant39/1 -> Bus Creator5/3  "VSM_HWAFastExitCons_OverrideTimeout"
  Bus Selector2/4 -> [RampDistance]  "<RampDistance>"
  If Action Subsystem1/1(Out1) -> Merge/2
  TrueDurationTime22/1 -> Compare To Constant121/1
  Logical Operator8/1 -> Bus Creator5/1  "VSM_HWAFastExitCons_ACCNotActive"
  Merge/1 -> Bus Selector2/1
  Compare To Constant44/1 -> Logical Operator8/3
  HOD/1 -> Bus Selector3/1
  Compare To Constant76/1 -> TrueDurationTime13/1
  Compare To Constant143/1 -> Bus Creator2/6  "VSM_HWASlowExitCons_TCS2Active3000ms"
  Constant8/1 -> If Action Subsystem1/4(In4)  "RampDistance"
  Logical Operator18/1 -> TrueDurationTime17/1
  Compare To Constant137/1 -> Logical Operator31/2
  HDCControl/1 -> Compare To Constant77/1
  If/1 -> If Action Subsystem/Action
  Compare To Constant77/1 -> TrueDurationTime24/1
  RampDistance/1 -> If Action Subsystem/4(RampDistance)
  Constant3/1 -> If Action Subsystem1/2(In2)  "FormOfWay"
  If/2 -> If Action Subsystem1/Action
  HWASubstate/3(TJAFastExit_b) -> TJAFastExit_b/1  "VSM_HWAFastExit_b"
  EHR_Switch1/1 -> If/1
  Constant10/1 -> If Action Subsystem1/5(In5)  "MapDataValid"
  Compare To Constant139/1 -> Bus Creator2/2  "VSM_HWASlowExitCons_MSRActive800ms"
  [HandsOn] -> Logical Operator30/2
  Compare To Constant121/1 -> Logical Operator33/1  "OverrideTimeout"
  [DrivingOnHighWay] -> Compare To Constant86/1
  Compare To Constant23/1 -> Logical Operator4/1
  Compare To Constant21/1 -> Logical Operator4/2
  Compare To Constant22/1 -> Logical Operator4/3
  [PilotSts] -> Compare To Constant23/1, Compare To Constant21/1, Compare To Constant22/1
  [HWAActive_b] -> Switch1/2
  Constant11/1 -> Switch1/3
  Switch2/1 -> Switch1/1
  Logical Operator4/1 -> Switch2/2
  Constant12/1 -> Switch2/1
  Constant14/1 -> Switch2/3
  Switch1/1 -> VSM_HWANOA_Mode/1  "VSM_HWANOA_Mode"
  ACCFailure/1 -> Compare To Constant24/1
  Compare To Constant24/1 -> Bus Creator2/11  "VSM_HWASlowExitCons_ACCError"
  Logical Operator1/1 -> HWASubstate/7(DoubleLineLost_b)
  Compare To Constant/1 -> Logical Operator1/1
  [VehicleSpd] -> Compare To Constant/1
  TJAError/1 -> [TJAError]  "VSM_Diagnostic_TJAError"
  [TJAError] -> HWASubstate/10(TJAError)
  Compare To Constant2/1 -> Bus Creator2/8  "VSM_HWASlowExitCons_HWAError_Inhibit"
  [HWAError] -> Compare To Constant3/1
  Compare To Constant3/1 -> Bus Creator/1
  [HWAError] -> Compare To Constant4/1
  Compare To Constant4/1 -> Bus Creator1/1

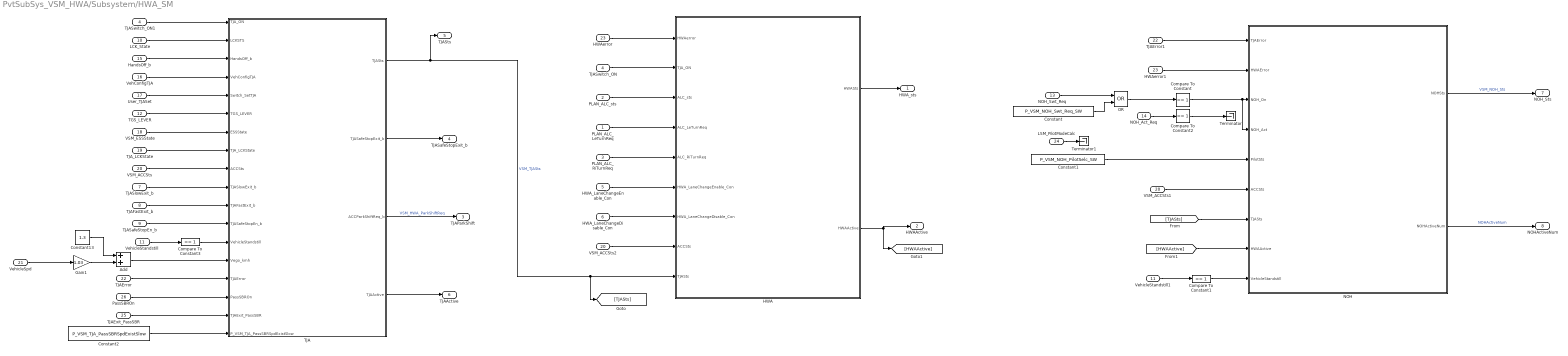
== system PvtSubSys_VSM_HWA/Subsystem/HWA_SM ==
  PLAN_ALC_LeTurnReq : Inport
  PLAN_ALC_sts : Inport  Port=2
  PLAN_ALC_RiTurnReq : Inport  Port=3
  TJASwitch_ON : Inport  Port=4
  HWA_LaneChangeEnable_Con : Inport  Port=5
  HWA_LaneChangeDisable_Con : Inport  Port=6
  TJASlowExit_b : Inport  Port=7
  TJAFastExit_b : Inport  Port=8
  TJASafeStopEn_b : Inport  Port=9
  LCK_State : Inport  Port=10
  VehicleStandstill : Inport  Port=11
  TGS_LEVER : Inport  Port=12
  NOH_Swt_Req : Inport  Port=13
  NOH_Act_Req : Inport  Port=14
  HandsOff_b : Inport  Port=15
  VehConfigTJA : Inport  Port=16
  User_TJASet : Inport  Port=17
  VSM_ESSState : Inport  Port=18
  TJA_LCKState : Inport  Port=19
  VSM_ACCSts : Inport  Port=20
  VehicleSpd : Inport  Port=21
  TJAError : Inport  Port=22
  HWAerror : Inport  Port=23
  LSM_PilotModeCalc : Inport  Port=24
  TJAExit_PassSBR : Inport  Port=25
  PassSBROn : Inport  Port=26
  Add : Sum  OutDataTypeStr=uint8
  Compare To Constant{,1..3} (4 alike) : simulink/Logic and Bit Operations/Compare To Constant  relop===  const=1  OutDataTypeStr=boolean
  Constant : Constant  Value=P_VSM_NOH_Swt_Req_SW
  Constant1 : Constant  Value=P_VSM_NOH_PilotSelc_SW
  Constant13 : Constant  Value=1.3
  Constant2 : Constant  Value=P_VSM_TJA_PassSBRSpdExistSlow
  Gain1 : Gain  Gain=1.03
  HWA : Stateflow chart  TreatAsAtomicUnit=on
  HWAerror1 : InportShadow  Port=23
  NOH : Stateflow chart  TreatAsAtomicUnit=on
  OR : Logic  Operator=OR  AllPortsSameDT=off  OutDataTypeStr=boolean
  TJA : Stateflow chart  TreatAsAtomicUnit=on
  TJAError1 : InportShadow  Port=22
  TJASwitch_ON1 : InportShadow  Port=4
  Terminator : Terminator
  Terminator1 : Terminator
  VSM_ACCSts1 : InportShadow  Port=20
  VSM_ACCSts2 : InportShadow  Port=20
  VehicleStandstill1 : InportShadow  Port=11
  HWA_sts : Outport
  HWAActive : Outport  Port=2
  TJAParkShift : Outport  Port=3
  TJASafeStopExit_b : Outport  Port=4
  TJASts : Outport  Port=5
  TJAActive : Outport  Port=6
  NOH_Sts : Outport  Port=7
  NOHActiveNum : Outport  Port=8
  wires:
  Constant2/1 -> TJA/18(P_VSM_TJA_PassSBRSpdExistSlow)
  TJAExit_PassSBR/1 -> TJA/17(TJAExit_PassSBR)
  PassSBROn/1 -> TJA/16(PassSBROn)
  NOH/2(NOHActiveNum) -> NOHActiveNum/1  "NOHActiveNum"
  LSM_PilotModeCalc/1 -> Terminator1/1
  Compare To Constant/1 -> NOH/3(NOH_On), NOH/4(NOH_Act)
  Compare To Constant2/1 -> Terminator/1
  Constant/1 -> OR/2
  NOH_Swt_Req/1 -> OR/1
  NOH_Act_Req/1 -> Compare To Constant2/1
  Compare To Constant1/1 -> NOH/9(VehicleStandstill)
  VehicleStandstill1/1 -> Compare To Constant1/1
  [HWAActive] -> NOH/8(HWAActive)
  [TJASts] -> NOH/7(TJASts)
  VSM_ACCSts1/1 -> NOH/6(ACCSts)
  HWAerror1/1 -> NOH/2(HWAError)
  TJAError1/1 -> NOH/1(TJAError)
  OR/1 -> Compare To Constant/1
  NOH/1(NOHSts) -> NOH_Sts/1  "VSM_NOH_Sts"
  Constant1/1 -> NOH/5(PilotSts)
  HWAerror/1 -> HWA/1(HWAerror)
  TJA/4(TJAActive) -> TJAActive/1
  VehicleSpd/1 -> Gain1/1
  Add/1 -> TJA/14(Vego_kmh)
  Gain1/1 -> Add/2
  Constant13/1 -> Add/1
  TJA/1(TJASts) -> TJASts/1, HWA/9(TJASts), [TJASts]  "VSM_TJASts"
  TJA/2(TJASafeStopExit_b) -> TJASafeStopExit_b/1
  TJA/3(ACCParkShiftReq_b) -> TJAParkShift/1  "VSM_HWA_ParkShiftReq"
  VSM_ACCSts/1 -> TJA/9(ACCSts)
  TJA_LCKState/1 -> TJA/8(TJA_LCKState)
  VSM_ESSState/1 -> TJA/7(ESSState)
  User_TJASet/1 -> TJA/5(Switch_SetTJA)
  VehConfigTJA/1 -> TJA/4(VehConfigTJA)
  HandsOff_b/1 -> TJA/3(HandsOff_b)
  Compare To Constant3/1 -> TJA/13(VehicleStandstill)
  TJAFastExit_b/1 -> TJA/11(TJAFastExit_b)
  TJASafeStopEn_b/1 -> TJA/12(TJASafeStopEn_b)
  TJASlowExit_b/1 -> TJA/10(TJASlowExit_b)
  TGS_LEVER/1 -> TJA/6(TGS_LEVER)
  LCK_State/1 -> TJA/2(LCKSTS)
  TJASwitch_ON1/1 -> TJA/1(TJA_ON)
  VSM_ACCSts2/1 -> HWA/8(ACCSts)
  TJASwitch_ON/1 -> HWA/2(TJA_ON)
  VehicleStandstill/1 -> Compare To Constant3/1
  HWA_LaneChangeDisable_Con/1 -> HWA/7(HWA_LaneChangeDisable_Con)
  HWA/2(HWAActive) -> HWAActive/1, [HWAActive]
  HWA/1(HWASts) -> HWA_sts/1
  HWA_LaneChangeEnable_Con/1 -> HWA/6(HWA_LaneChangeEnable_Con)
  PLAN_ALC_RiTurnReq/1 -> HWA/5(ALC_RiTurnReq)
  PLAN_ALC_LeTurnReq/1 -> HWA/4(ALC_LeTurnReq)
  PLAN_ALC_sts/1 -> HWA/3(ALC_sts)
  TJAError/1 -> TJA/15(TJAError)

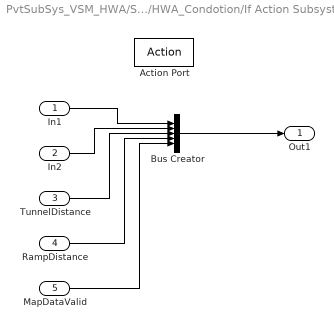
== system PvtSubSys_VSM_HWA/Subsystem/HWA_Condotion/If Action Subsystem ==
  In1 : Inport
  In2 : Inport  Port=2
  TunnelDistance : Inport  Port=3
  RampDistance : Inport  Port=4
  MapDataValid : Inport  Port=5
  Action Port : ActionPort
  Bus Creator : BusCreator  Inputs=5
  Out1 : Outport
  wires:
  In1/1 -> Bus Creator/1
  In2/1 -> Bus Creator/2
  Bus Creator/1 -> Out1/1
  TunnelDistance/1 -> Bus Creator/3
  RampDistance/1 -> Bus Creator/4
  MapDataValid/1 -> Bus Creator/5

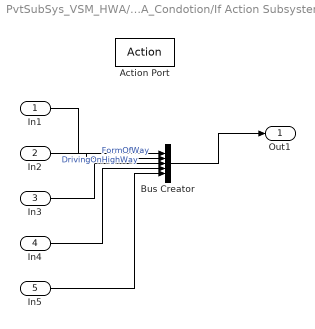
== system PvtSubSys_VSM_HWA/Subsystem/HWA_Condotion/If Action Subsystem1 ==
  In1 : Inport
  In2 : Inport  Port=2
  In3 : Inport  Port=3
  In4 : Inport  Port=4
  In5 : Inport  Port=5
  Action Port : ActionPort
  Bus Creator : BusCreator  Inputs=5
  Out1 : Outport
  wires:
  Bus Creator/1 -> Out1/1
  In2/1 -> Bus Creator/2  "FormOfWay"
  In1/1 -> Bus Creator/1  "DrivingOnHighWay"
  In3/1 -> Bus Creator/3
  In4/1 -> Bus Creator/4
  In5/1 -> Bus Creator/5

== stateflow chart PvtSubSys_VSM_HWA/Subsystem/HWA_Condotion/HWASubstate ==
  settings: executeAtInitialization=1
  state SlowExit [parallel]
    settings: executionOrder=1
    state Act
      en:
      TJASlowExit_b=0;
    state Warn
      en:
      TJASlowExit_b=1;
    (default) -> Act
    Act -> Warn : [(TJASts==3)&&...
        | (TJASlowExitConditions_b)]
    Warn -> Act : [TJASts~=3 && TJASts~=9 && TJASts~=10]
        | %TJA 非Active
  state Main [parallel]
    settings: executionOrder=2
    state Exit
      en:
      HWAWarningLevel=0;
      TJASafeStopEn_b=false;
      TJAFastExit_b=true;
    state ActiveWaitting
      en:
      TJASafeStopEn_b=false;
      TJAFastExit_b=false;
    state P
      state Active
        en:
        Cnt=0;
        HWAWarningLevel=0;
        TJASafeStopEn_b=false;
        TJAFastExit_b=false;
      state Warning1
        en:
        TJASafeStopEn_b=false;
        TJAFastExit_b=false;
        Cnt=0;
        du:
        Cnt=min(300,Cnt+1);
        state Warning1Suppress1_Drow
          en:
          HWAWarningLevel=0;
          Cnt1=0;
          Cnt2=0;
          Cnt3=0;
          du:
          Cnt3=min(4000,Cnt3+1);
          ex:
          Cnt3=0;
        state Warning1Suppress
          en:
          HWAWarningLevel=0;
          Cnt1=0;
          Cnt2=0;
          Cnt3=0;
          du:
          Cnt2=min(600,Cnt2+1);
          ex:
          Cnt2=0;
        state Warning1Active
          en:
          HWAWarningLevel=1;
          Cnt1=0;
          Cnt2=0;
          Cnt3=0;
          du:
          Cnt1=min(300,Cnt1+1);
        (default) -> Warning1Active
        Warning1Suppress -> Warning1Active : [Cnt2>500]
        Warning1Suppress1_Drow -> Warning1Active : [Cnt3>3000]
        Warning1Active -> Warning1Suppress [order 2] : [Cnt1>150&&DriverSts==2]
        Warning1Active -> Warning1Suppress1_Drow [order 1] : [Cnt1>150&&DriverSts==6]
      state Warning2
        en:
        TJASafeStopEn_b=false;
        TJAFastExit_b=false;
        Cnt=0;
        du:
        Cnt=min(300,Cnt+1);
        state Warning2Suppress
          en:
          HWAWarningLevel=0;
          Cnt1=0;
          Cnt2=0;
          Cnt3=0;
          du:
          Cnt2=min(600,Cnt2+1);
          ex:
          Cnt2=0;
        state Warning2Suppress_Drow
          en:
          HWAWarningLevel=0;
          Cnt1=0;
          Cnt2=0;
          Cnt3=0;
          du:
          Cnt3=min(4000,Cnt3+1);
          ex:
          Cnt3=0;
        state Warning2Active
          en:
          HWAWarningLevel=2;
          Cnt1=0;
          Cnt2=0;
          Cnt3=0;
          du:
          Cnt1=min(300,Cnt1+1);
        (default) -> Warning2Active
        Warning2Suppress_Drow -> Warning2Active : [Cnt3>3000]
        Warning2Suppress -> Warning2Active : [Cnt2>500]
        Warning2Active -> Warning2Suppress [order 2] : [Cnt1>200&&DriverSts==3]
        Warning2Active -> Warning2Suppress_Drow [order 1] : [Cnt1>200&&DriverSts==7]
      state Warning3
        en:
        TJASafeStopEn_b=false;
        TJAFastExit_b=false;
        Cnt=0;
        du:
        Cnt=min(300,Cnt+1);
        state Warning3Suppress_Drow
          en:
          HWAWarningLevel=0;
          Cnt1=0;
          Cnt2=0;
          Cnt3=0;
          du:
          Cnt3=min(4000,Cnt3+1);
          ex:
          Cnt3=0;
        state Warning3Suppress
          en:
          HWAWarningLevel=0;
          Cnt1=0;
          Cnt2=0;
          Cnt3=0;
          du:
          Cnt2=min(600,Cnt2+1);
          ex:
          Cnt2=0;
        state Warning3Active
          en:
          HWAWarningLevel=3;
          Cnt1=0;
          Cnt2=0;
          Cnt3=0;
          du:
          Cnt1=min(300,Cnt1+1);
        (default) -> Warning3Active
        Warning3Suppress -> Warning3Active : [Cnt2>500]
        Warning3Suppress_Drow -> Warning3Active : [Cnt3>3000]
        Warning3Active -> Warning3Suppress [order 2] : [Cnt1>250&&DriverSts==4]
        Warning3Active -> Warning3Suppress_Drow [order 1] : [Cnt1>250&&DriverSts==8]
      (default) -> Active
      Active -> Warning1 [order 3] : [((HandsOff_b)&&...
          | (in(SlowExit.Warn)))||...
          | (DriverSts==2)||...
          | (DriverSts==6)||...
          | (HandsOffWarnLevel==1)]
      Warning1 -> Active [order 3] : [(in(SlowExit.Act))&&...
          | (DriverSts==1)&&...
          | (Cnt2==0)&&(Cnt3==0)&&...
          | (HandsOffWarnLevel==0)]
      Active -> Warning2 [order 2] : [(DriverSts==3)||...
          | (DriverSts==7)]
      Warning2 -> Active [order 3] : [(in(SlowExit.Act))&&...
          | (DriverSts==1)&&...
          | (HandsOffWarnLevel==0)]
      Active -> Warning3 [order 1] : [(DriverSts==4)||...
          | (DriverSts==8)]
      Warning3 -> Active [order 4] : [(in(SlowExit.Act))&&...
          | (DriverSts==1)&&...
          | (HandsOffWarnLevel==0)]
      Warning3 -> Warning1 [order 7] : [(in(SlowExit.Act))&&...
          | (DriverSts==1)&&...
          | (Cnt2==0)&&(Cnt3==0)&&...
          | (HandsOffWarnLevel==1)]
      Warning1 -> Warning3 [order 1] : [(DriverSts==4)||...
          | (DriverSts==8)]
      Warning3 -> Warning1 [order 3] : [(in(SlowExit.Act))&&...
          | ((DriverSts==2)||...
          | (DriverSts==6))&&...
          | (Cnt2==0)&&(Cnt3==0)&&...
          | (HandsOffWarnLevel<=1)]
      Warning1 -> Warning2 [order 2] : [((HandsOff_b)&&...
          | (in(SlowExit.Warn))&&...
          | (Cnt>150))||...
          | (DriverSts==3)||...
          | (DriverSts==7)||...
          | (HandsOffWarnLevel==2)]
      Warning2 -> Warning1 [order 2] : [(in(SlowExit.Act))&&...
          | ((DriverSts==2)||...
          | (DriverSts==6))&&...
          | (Cnt2==0)&&(Cnt3==0)&&...
          | (HandsOffWarnLevel<=1)]
      Warning2 -> Warning1 [order 4] : [(in(SlowExit.Act))&&...
          | (DriverSts==1)&&...
          | (Cnt2==0)&&(Cnt3==0)&&...
          | (HandsOffWarnLevel==1)]
      Warning3 -> Warning2 [order 5] : [(in(SlowExit.Act))&&...
          | ((DriverSts==2)||...
          | (DriverSts==6))&&...
          | (Cnt2==0)&&(Cnt3==0)&&...
          | (HandsOffWarnLevel==2)]
      Warning2 -> Warning3 [order 1] : [((HandsOff_b)&&...
          | (in(SlowExit.Warn))&&...
          | (Cnt>200))||...
          | (DriverSts==4)||...
          | (DriverSts==8)||...
          | (HandsOffWarnLevel==3)]
      Warning3 -> Warning2 [order 2] : [(in(SlowExit.Act))&&...
          | ((DriverSts==3)||...
          | (DriverSts==7))&&...
          | (Cnt2==0)&&(Cnt3==0)&&...
          | (HandsOffWarnLevel<=2)]
      Warning3 -> Warning2 [order 6] : [(in(SlowExit.Act))&&...
          | (DriverSts==1)&&...
          | (Cnt2==0)&&(Cnt3==0)&&...
          | (HandsOffWarnLevel==2)]
    state SafeStop
      en:
      Cnt=0;
      HWAWarningLevel=4;
      TJASafeStopEn_b=true;
      TJAFastExit_b=false;
    (default) -> ActiveWaitting
    Exit -> ActiveWaitting : [(TJASts~=3 && TJASts~=9 && TJASts~=10)]
    ActiveWaitting -> P : [TJASts==3]
    P -> ActiveWaitting [order 3] : [TJASts~=3 && TJASts~=9 && TJASts~=10]
    P -> Exit [order 1] : [((HandsOn_b)&&...
        | ((in(SlowExit.Warn))))||...
        | SomeHWASafeStop2ExitConditions_b]
    Warning3 -> SafeStop [order 1] : [(HandsOff_b)&&...
        | (in(SlowExit.Warn))&&...
        | (Cnt>250)]
    P -> SafeStop [order 2] : [(DoubleLineLost_b&&TJALineValid==0&&HandsOff_b)||...
        | (DriverSts==5)||...
        | (DriverSts==9)||...
        | (HandsOffWarnLevel==4)||...
        | (((TJAError==1))&&(HandsOff_b))]
    SafeStop -> Exit : [SomeHWASafeStop2ExitConditions_b||...
        | (HandsOn_b&&(DriverSts!=5)&&(DriverSts!=9)&&(DriverSts!=0))||...
        | (HandsOn_b&&(DriverSts==0))]
  data: SomeHWASafeStop2ExitConditions_b input boolean; TJASlowExitConditions_b input boolean; HandsOn_b input boolean; HandsOff_b input boolean; HWAWarningLevel output uint8 =0; TJASafeStopEn_b output boolean =false; TJAFastExit_b output boolean =false; Cnt local double size=1 [0..500] =0; DriverSts input; HandsOffWarnLevel input; Cnt1 local double size=1 [0..500] =0; Cnt2 local double size=1 [0..500] =0; TJASlowExit_b output boolean =false; Cnt3 local double; DoubleLineLost_b input boolean; TJALineValid input boolean; TJASts input double; TJAError input uint8
